simulink model "SPMe_CC_simulink"  (R2024a)
settings: Solver=FixedStepAuto  StartTime=0.0  StopTime=t_end  FixedStep=dt  MaxStep=1  RelTol=1e-6
values from neighbouring files (symbols this model uses):
  alpha = 64.526    [EqCM.m]
  I = 4.6*C_rates(c)    [run_SPMe_fast_discharge.m]    (also in run_SPMe_sweep.m; run_SPMe_vent.m = squeeze(sol.I.Data))
  T_amb = 273.15+25    (= 298.15)    [EqCM.m]    (also in run_SPMe_vent.m = param.T_amb)
  V_min = 0    [run_SPMe_fast_discharge.m]    (also in run_SPMe_sweep.m = 3; run_SPMe_vent.m = -3)
undefined symbols (not defined in the file or in its folder): A, DMC, E_p, EC, L_p0, m_an, M_C6, P_atm, P_crit, R, sigma_0, V_head_0, x_sei_0, y_dmc, y_ec
libraries: simulink x1
settings Model: Creator=tom  LastModifiedBy=Vivian
settings SolverCC: AlgebraicLoopSolver=TrustRegion
settings DebuggingCC: UnconnectedInputMsg=warning  UnconnectedOutputMsg=warning  UnconnectedLineMsg=warning
settings ModelReferenceCC: EnableRefExpFcnMdlSchedulingChecks=on
settings RTWCC: GPUComputeCapability=3.5  DLArmComputeVersion=19.05

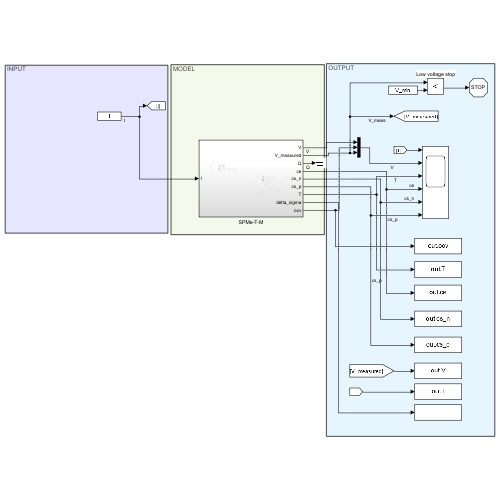
[thumbnail: Simulink's stored preview of the top-level diagram]
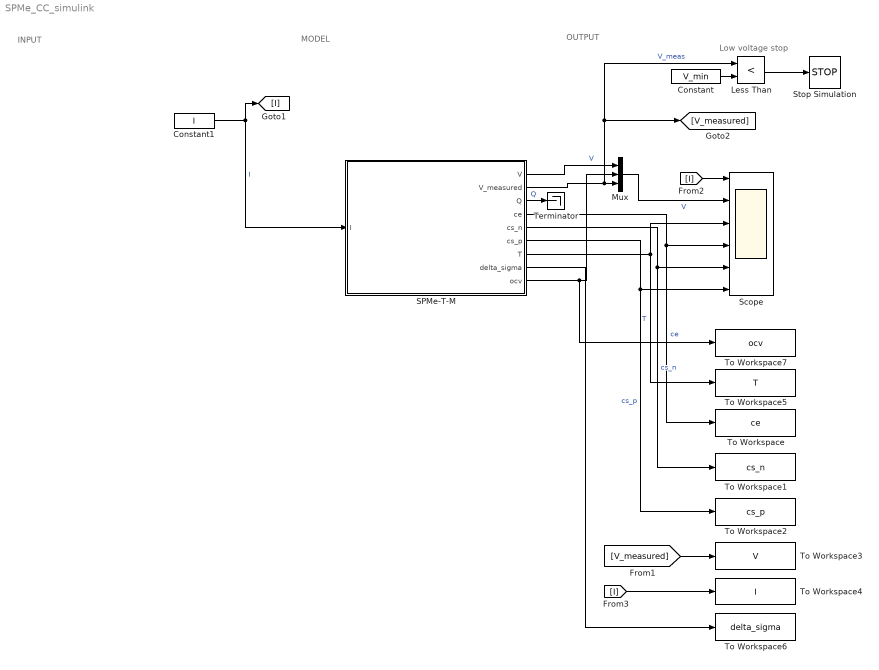
== system SPMe_CC_simulink ==
  note: OUTPUT
  note: MODEL
  note: INPUT
  note: Low voltage stop
  Constant : Constant  Value=V_min
  Constant1 : Constant  Value=I
  Less Than : RelationalOperator  Operator=<  OutDataTypeStr=boolean  RndMeth=Simplest  InputSameDT=off
  Mux : Mux  Inputs=3
  SPMe-T-M : Subsystem
  Scope : Scope  NumInputPorts=6
  Stop Simulation : Stop
  Terminator : Terminator
  To Workspace : ToWorkspace  VariableName=ce  SaveFormat=Timeseries  SampleTime=-1
  To Workspace1 : ToWorkspace  VariableName=cs_n  SaveFormat=Timeseries  SampleTime=-1
  To Workspace2 : ToWorkspace  VariableName=cs_p  SaveFormat=Timeseries  SampleTime=-1
  To Workspace3 : ToWorkspace  VariableName=V  SaveFormat=Timeseries  SampleTime=-1
  To Workspace4 : ToWorkspace  VariableName=I  SaveFormat=Timeseries  SampleTime=-1
  To Workspace5 : ToWorkspace  VariableName=T  SaveFormat=Timeseries  SampleTime=-1
  To Workspace6 : ToWorkspace  VariableName=delta_sigma  SaveFormat=Timeseries  SampleTime=-1
  To Workspace7 : ToWorkspace  VariableName=ocv  SaveFormat=Timeseries  SampleTime=-1
  wires:
  SPMe-T-M/5(cs_n) -> To Workspace1/1, Scope/5  "cs_n"
  SPMe-T-M/6(cs_p) -> To Workspace2/1, Scope/6  "cs_p"
  Less Than/1 -> Stop Simulation/1
  Constant/1 -> Less Than/2
  SPMe-T-M/4(ce) -> To Workspace/1, Scope/4  "ce"
  SPMe-T-M/1(V) -> Mux/1  "V"
  SPMe-T-M/2(V_measured) -> Less Than/1, [V_measured], Mux/3  "V_meas"
  Constant1/1 -> SPMe-T-M/1(I), [I]  "I"
  Mux/1 -> Scope/2  "V"
  [V_measured] -> To Workspace3/1
  [I] -> Scope/1
  [I] -> To Workspace4/1
  SPMe-T-M/8(delta_sigma) -> To Workspace6/1
  SPMe-T-M/3(Q) -> Terminator/1  "Q"
  SPMe-T-M/7(T) -> To Workspace5/1, Scope/3  "T"
  SPMe-T-M/9(ocv) -> Mux/2, To Workspace7/1

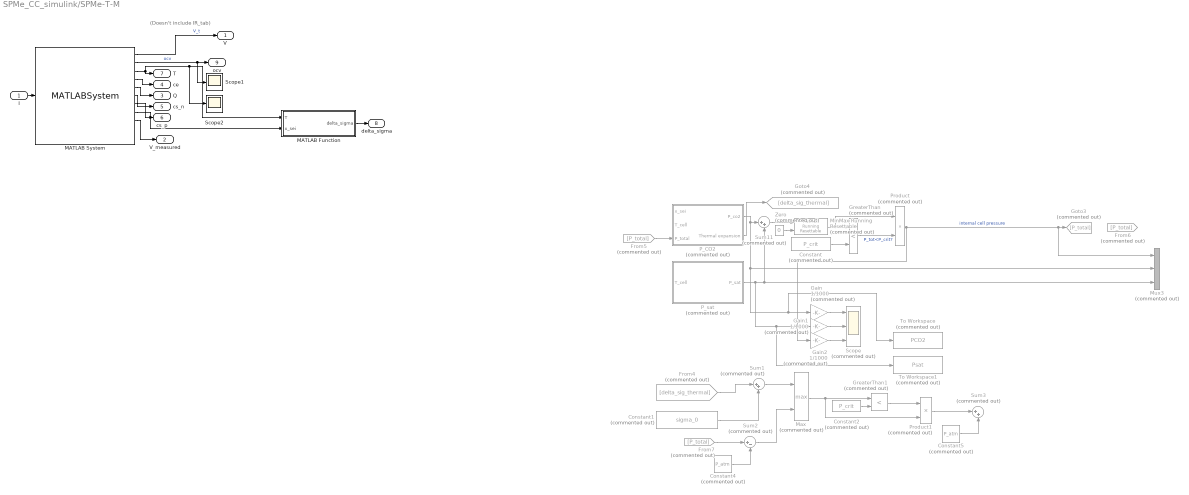
== system SPMe_CC_simulink/SPMe-T-M ==
  note: (Doesn't include IR_tab)
  I : Inport
  Constant : Constant  Commented=on  Value=P_crit
  Constant1 : Constant  Commented=on  Value=sigma_0
  Constant2 : Constant  Commented=on  Value=P_crit
  Constant4 : Constant  Commented=on  Value=P_atm
  Constant5 : Constant  Commented=on  Value=P_atm
  From4 : From  Commented=on  GotoTag=delta_sig_thermal
  From5 : From  Commented=on  GotoTag=P_total
  From6 : From  Commented=on  GotoTag=P_total
  From7 : From  Commented=on  GotoTag=P_total
  Gain : Gain  Commented=on  Gain=1/1000
  Gain1 : Gain  Commented=on  Gain=1/1000
  Gain2 : Gain  Commented=on  Gain=1/1000
  Goto3 : Goto  Commented=on  GotoTag=P_total
  Goto4 : Goto  Commented=on  GotoTag=delta_sig_thermal
  GreaterThan : RelationalOperator  Commented=on  Operator=<  OutDataTypeStr=boolean  RndMeth=Simplest  InputSameDT=off
  GreaterThan1 : RelationalOperator  Commented=on  Operator=<  OutDataTypeStr=boolean  RndMeth=Simplest  InputSameDT=off
  MATLAB Function : MATLAB Function  TreatAsAtomicUnit=on
  MATLAB System : MATLABSystem  System=pybamm_bat  SimulateUsing=Interpreted execution
      mask Type: pybamm_bat
      mask Display:
      | disp('pybamm_bat');
      | port_label('input',1,'current');
      | port_label('output',1,'V_t');
      | port_label('output',2,'ocv');
      | port_label('output',3,'T');
      | port_label('output',4,'ce');
      | port_label('output',5,'heating');
      | port_label('output',6,'neg_conc');
      | port_label('output',7,'pos_conc');
      | port_label('output',8,'x_sei');
      | port_label('output',9,'V_meas');
      | port_label('output',10,'ocp_n');
      | port_label('output',11,'ocp_p');
  Max : MinMax  Commented=on  Function=max  Inputs=2
  MinMax Running Resettable : simulink/Math Operations/MinMax Running Resettable  Commented=on  Function=max  vinit=0
  Mux3 : Mux  Commented=on  Inputs=3
  P_CO2 : Subsystem  Commented=on
  P_sat : Subsystem  Commented=on
  Product : Product  Commented=on
  Product1 : Product  Commented=on
  Scope : Scope  Commented=on  NumInputPorts=3
  Scope1 : Scope
  Scope2 : Scope
  Sum1 : Sum  Commented=on  Inputs=|++
  Sum11 : Sum  Commented=on  Inputs=|++
  Sum2 : Sum  Commented=on  Inputs=|+-
  Sum3 : Sum  Commented=on  Inputs=|++
  To Workspace : ToWorkspace  Commented=on  VariableName=PCO2  SaveFormat=Timeseries  SampleTime=-1
  To Workspace1 : ToWorkspace  Commented=on  VariableName=Psat  SaveFormat=Timeseries  SampleTime=-1
  Zero : Constant  Commented=on  Value=0  OutDataTypeStr=Inherit: Inherit via back propagation
  V : Outport
  V_measured : Outport  Port=2
  Q : Outport  Port=3  VectorParamsAs1DForOutWhenUnconnected=off
  ce : Outport  Port=4
  cs_n : Outport  Port=5  VectorParamsAs1DForOutWhenUnconnected=off
  cs_p : Outport  Port=6  VectorParamsAs1DForOutWhenUnconnected=off
  T : Outport  Port=7
  delta_sigma : Outport  Port=8
  ocv : Outport  Port=9
  wires:
  MATLAB System/4 -> ce/1
  MATLAB System/5 -> Q/1
  MATLAB System/6 -> cs_n/1
  MATLAB System/7 -> cs_p/1
  MATLAB System/1 -> V/1  "V_t"
  MATLAB System/9 -> V_measured/1
  MATLAB System/2 -> Scope1/1, ocv/1  "ocv"
  I/1 -> MATLAB System/1
  MATLAB System/3 -> T/1, MATLAB Function/1(T), Scope2/1
  From7/1 -> Sum2/1
  Sum11/1 -> MinMax Running Resettable/1
  Zero/1 -> MinMax Running Resettable/2
  GreaterThan/1 -> Product/2  "P_tot<P_crit?"
  Gain2/1 -> Scope/3
  Constant1/1 -> Sum1/2
  Constant4/1 -> Sum2/2
  Constant/1 -> GreaterThan/2
  Sum1/1 -> Max/1
  Constant2/1 -> GreaterThan1/2
  P_sat/1(P_sat) -> To Workspace1/1, Gain1/1, Sum11/2, Mux3/3
  Constant5/1 -> Sum3/2
  MinMax Running Resettable/1 -> Product/1, GreaterThan/1
  Product1/1 -> Sum3/1
  From4/1 -> Sum1/1
  Gain/1 -> Scope/1
  From5/1 -> P_CO2/3(P_total)
  Product/1 -> Gain2/1, Mux3/1, Goto3/1  "internal cell pressure"
  Max/1 -> GreaterThan1/1, Product1/2
  Gain1/1 -> Scope/2
  GreaterThan1/1 -> Product1/1
  P_CO2/1(P_co2) -> To Workspace/1, Gain/1, Mux3/2, Sum11/1
  P_CO2/2(Thermal expansion) -> Goto4/1
  Sum2/1 -> Max/2
  MATLAB System/8 -> MATLAB Function/2(x_sei)
  MATLAB Function/1(delta_sigma) -> delta_sigma/1

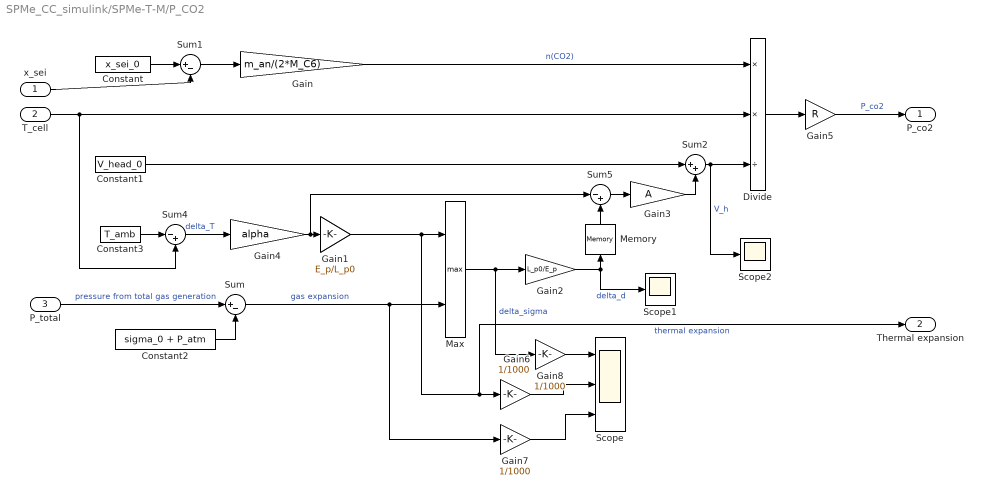
== system SPMe_CC_simulink/SPMe-T-M/P_CO2 ==
  x_sei : Inport
  T_cell : Inport  Port=2
  P_total : Inport  Port=3
  Constant : Constant  Value=x_sei_0
  Constant1 : Constant  Value=V_head_0
  Constant2 : Constant  Value=sigma_0 + P_atm
  Constant3 : Constant  Value=T_amb
  Divide : Product  Inputs=**/
  Gain : Gain  Gain=m_an/(2*M_C6)
  Gain1 : Gain  Gain=E_p/L_p0
  Gain2 : Gain  Gain=L_p0/E_p
  Gain3 : Gain  Gain=A
  Gain4 : Gain  Gain=alpha
  Gain5 : Gain  Gain=R
  Gain6 : Gain  Gain=1/1000
  Gain7 : Gain  Gain=1/1000
  Gain8 : Gain  Gain=1/1000
  Max : MinMax  Function=max  Inputs=2
  Memory : Memory
  Scope : Scope  NumInputPorts=3
  Scope1 : Scope
  Scope2 : Scope
  Sum : Sum  Inputs=|+-
  Sum1 : Sum  Inputs=|+-
  Sum2 : Sum  Inputs=|++
  Sum4 : Sum  Inputs=|-+
  Sum5 : Sum  Inputs=|-+
  P_co2 : Outport
  Thermal expansion : Outport  Port=2
  wires:
  Sum4/1 -> Gain4/1  "delta_T"
  Gain2/1 -> Scope1/1, Memory/1  "delta_d"
  Constant1/1 -> Sum2/1
  Sum1/1 -> Gain/1
  T_cell/1 -> Divide/2, Sum4/2
  Divide/1 -> Gain5/1
  Sum5/1 -> Gain3/1
  Max/1 -> Gain8/1, Gain2/1  "delta_sigma"
  Gain4/1 -> Sum5/1, Gain1/1
  Gain5/1 -> P_co2/1  "P_co2"
  Constant/1 -> Sum1/1
  Gain3/1 -> Sum2/2
  Gain/1 -> Divide/1  "n(CO2)"
  Sum2/1 -> Scope2/1, Divide/3  "V_h"
  Constant3/1 -> Sum4/1
  x_sei/1 -> Sum1/2
  Gain7/1 -> Scope/3
  Gain1/1 -> Thermal expansion/1, Gain6/1, Max/1  "thermal expansion"
  Memory/1 -> Sum5/2
  Sum/1 -> Gain7/1, Max/2  "gas expansion"
  P_total/1 -> Sum/1  "pressure from total gas generation"
  Constant2/1 -> Sum/2
  Gain6/1 -> Scope/2
  Gain8/1 -> Scope/1

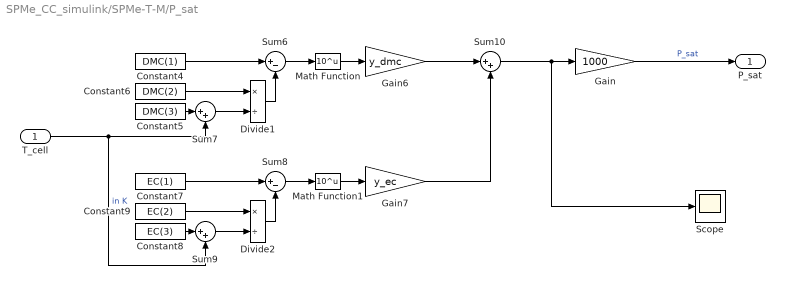
== system SPMe_CC_simulink/SPMe-T-M/P_sat ==
  T_cell : Inport
  Constant4 : Constant  Value=DMC(1)
  Constant5 : Constant  Value=DMC(3)
  Constant6 : Constant  Value=DMC(2)
  Constant7 : Constant  Value=EC(1)
  Constant8 : Constant  Value=EC(3)
  Constant9 : Constant  Value=EC(2)
  Divide1 : Product  Inputs=*/
  Divide2 : Product  Inputs=*/
  Gain : Gain  Gain=1000
  Gain6 : Gain  Gain=y_dmc
  Gain7 : Gain  Gain=y_ec
  Math Function : Math  Operator=10^u
  Math Function1 : Math  Operator=10^u
  Scope : Scope
  Sum10 : Sum  Inputs=|++
  Sum6 : Sum  Inputs=|+-
  Sum7 : Sum  Inputs=|++
  Sum8 : Sum  Inputs=|+-
  Sum9 : Sum  Inputs=|++
  P_sat : Outport
  wires:
  Constant7/1 -> Sum8/1
  Math Function1/1 -> Gain7/1
  Sum9/1 -> Divide2/2
  Sum6/1 -> Math Function/1
  Sum7/1 -> Divide1/2
  Divide2/1 -> Sum8/2
  T_cell/1 -> Sum9/2, Sum7/2  "in K"
  Constant4/1 -> Sum6/1
  Math Function/1 -> Gain6/1
  Constant8/1 -> Sum9/1
  Sum8/1 -> Math Function1/1
  Constant9/1 -> Divide2/1
  Divide1/1 -> Sum6/2
  Constant5/1 -> Sum7/1
  Constant6/1 -> Divide1/1
  Gain6/1 -> Sum10/1
  Gain7/1 -> Sum10/2
  Sum10/1 -> Scope/1, Gain/1
  Gain/1 -> P_sat/1  "P_sat"

== matlab function SPMe_CC_simulink/SPMe-T-M/MATLAB Function ==
  data: T input; x_sei input; delta_sigma output
function delta_sigma  = expansion(T,x_sei)
%XSEI2PTOTAL 
% Mechanical params
M_C6 = 72/1000; %kg/mol
% V_head_0 = 6.65e-6; %m3 (0.121*0.074*0.0055)*0.135
% L = 2.4/1000; %m
% E = 0.19e6; %Pa
% alpha_cell = 1.1e-6; %m/K
% P_atm = 101; %kPa
% P_crit = 158.7731; %kPa
R = 8.3145; %J.mol-1.K-1
A = 0.009; %m2 (0.121*0.074)
DMC = [6.4338; 1413; -44.25]; %Antoine coeffs [A B C] 
EC = [6.4897; 1836.57; -102.23];
y_dmc = 0.7;
y_ec = 1-y_dmc;         
m_an = 0.0191; 
x_sei_0 = 0.15;
% T_amb = 273.15+25; % K
% sigma_0 = 1.5120e+04;

% Internal cell pressure
V_head_0 = 6.65e-06; %m-3
L_p0 = 2.4e-3; %m for 2 poron
E_p = 0.19e6; %Pa Young's modulus for poron
% E_c = 1e12; %assume large by default
alpha = 1.1e-6; %m/K
P_atm = 101e3; %Pa
% P_crit = 158e3; %Pa
% P0 = 14e3; %Pa
R = 8.3145; %J.mol-1.K-1
% k_b = 1.380649e-23; %m2.kg.s-2.K-1;
T_amb = 273.15+25; % K
sigma_0 = 1.5120e+04;
% L_cs0 = 5.5e-3; %m initial cell solid thickness
% V_cell = 0.130*0.089*0.055; % [130mm×89mm×5.5mm] active material

% P_elyte
Psat_EC = 10.^(EC(1)-EC(2)./(EC(3)+T));
Psat_DMC = 10.^(DMC(1)-DMC(2)./(DMC(3)+T)); 
P_elyte = (y_dmc*Psat_DMC + y_ec*Psat_EC)*1e3; 

% P_CO2
n_CO2 = 0.5*m_an/M_C6*(x_sei_0-x_sei);

% Solve for gas volume and pressure
delta_sigma_calc = P_elyte - sigma_0 - P_atm;
a = 1;
b = -(V_head_0 + A.*(L_p0/E_p*(delta_sigma_calc) - alpha.*(T-T_amb)));
c = -A*L_p0/E_p.*n_CO2.*R.*(T);
V_g0 = (-b+sqrt(max(b.^2-4.*a.*c,0)))/(2*a);
V_g = max(V_g0, V_head_0); % min V_g = V_head_0

P_CO2 = n_CO2.*R.*T./V_g;
P_gas = P_elyte + P_CO2;

delta_sigma = max(P_gas-P_atm-sigma_0, E_p./L_p0.*alpha.*(T-T_amb));
end
